simulink model "problem_4_2_simulink"  (R2017b)
settings: Solver=VariableStepAuto  StartTime=0.0  StopTime=20.0  RelTol=1e-3
settings Model: Creator=52938  LastModifiedBy=ghost
settings CodeAppCC: StateflowObjectComments=on

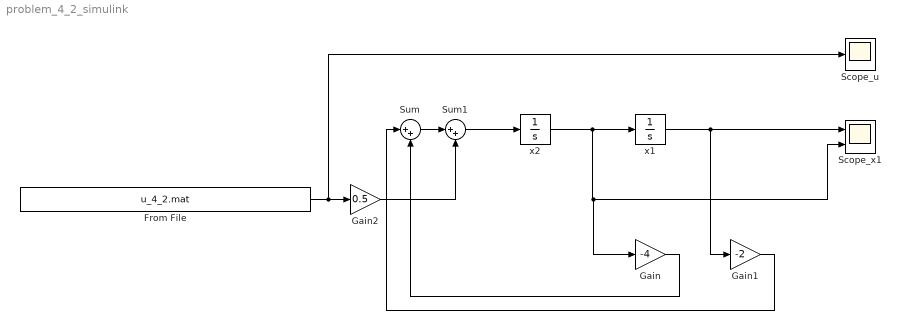
== system problem_4_2_simulink ==
  From File : FromFile  FileName=u_4_2.mat  SampleTime=0
  Gain : Gain  Gain=-4
  Gain1 : Gain  Gain=-2
  Gain2 : Gain  Gain=0.5
  Scope_u : Scope
  Scope_x1 : Scope  NumInputPorts=2
  Sum : Sum  Inputs=|++
  Sum1 : Sum  Inputs=|++
  x1 : Integrator  InitialCondition=-0.5
  x2 : Integrator
  wires:
  x1/1 -> Gain1/1, Scope_x1/1
  x2/1 -> Scope_x1/2, Gain/1, x1/1
  Gain/1 -> Sum/2
  Gain1/1 -> Sum/1
  Sum/1 -> Sum1/1
  From File/1 -> Scope_u/1, Gain2/1
  Sum1/1 -> x2/1
  Gain2/1 -> Sum1/2
